simulink model "RudderActuatorChannel_control_arx"  (R2015a)
settings: Solver=ode4  StartTime=0.0  StopTime=2.999  FixedStep=sampleTime  MaxStep=1e-3  MinStep=1e-4
undefined symbols (not defined in the file or in its folder): Acv, Aleak1, Aleak2, Aleak3, Aleak4, Aleak5, Aleakext, Aleakint, Ap, Ap_seal, Ar_seal, As_ehsv, Bkp_seal, Bp1, C, Cd, ControlTopology, DeltaQ_ehsv, EHSV, EHSV_Step, EHSVFreqTest, EHSVTest, ent_air, frictionstribeck_velocity, i_ehsv, Imax, K2_ehsv, K3_ehsv, K_Supply1, Ka1, Kd, Ki, Ki_ehsv, Kp, Kr_ehsv, ksi_ehsv, Kst, Kst_Enable, Kw_ehsv, L0, Load_cmd, Lp_seal, Lr_seal, Max_Cmd, Max_Load_TED, Max_Load_TEU, Min_Cmd, Mp1, ON_OFF_hyst, P10, Pcvac, Pcvi, Pcvr, Ps0, Pt0, Ql_ehsv, R, Rate_Limit, Return_Pressure, Rho ... (+24)
undefined symbols (not defined in the file): dpLVDT, Kd_N, ramLVDT, StateControl, xvLVDT
libraries: simulink x3
(part 2 of 2)

== system RudderActuatorChannel_control_arx/Actuation System/Actuator/Valves Dynamics/EHSV/EHSV 1st Stage ==
  i : Inport
  Add : Sum  Inputs=|+-
  Armature flapper : TransferFcn  Numerator=[1/Kr_ehsv]  Denominator=[1/(w_n_ehsv^2) 2*ksi_ehsv/w_n_ehsv 1]
  EHSV 1st stage test : TransferFcn  Numerator=[.001852*730^2]  Denominator=[1 2*0.4*730 730^2]
  Feedback wire : Gain  Gain=Kw_ehsv
  Flapper displacement at nozzles : Saturate  UpperLimit=xf_ehsv  LowerLimit=-xf_ehsv
  Hydraulic Amplifier : Gain  Gain=K2_ehsv
  "Hydraulic Amplifier Differential flow " : Saturate  UpperLimit=DeltaQ_ehsv  LowerLimit=-DeltaQ_ehsv
  Scope : Scope  NumInputPorts=2
      settings: TimeRange=2.999  YMin=-5~-5  YMax=5~5  SaveName=ScopeData3
  Servovalve control flow : Saturate  UpperLimit=Ql_ehsv  LowerLimit=-Ql_ehsv
  Spool : TransferFcn  Denominator=[As_ehsv 0]
  Spool displacement : Saturate  UpperLimit=xs_ehsv  LowerLimit=-xs_ehsv
  Spool Flow Gain : Gain  Gain=K3_ehsv
  Terminator : Terminator
  Torque motor : Gain  Gain=Ki_ehsv
  Torque motor current : Saturate  UpperLimit=i_ehsv  LowerLimit=-i_ehsv
  Xv : Outport
  wires:
  Torque motor/1 -> Add/1
  Feedback wire/1 -> Add/2
  i/1 -> EHSV 1st stage test/1, Torque motor current/1
  Armature flapper/1 -> Flapper displacement at nozzles/1
  Spool/1 -> Scope/1, Spool displacement/1
  Hydraulic Amplifier/1 -> "Hydraulic Amplifier Differential flow "/1
  Add/1 -> Armature flapper/1
  Flapper displacement at nozzles/1 -> Hydraulic Amplifier/1
  "Hydraulic Amplifier Differential flow "/1 -> Spool/1
  Spool displacement/1 -> Spool Flow Gain/1, Xv/1, Feedback wire/1
  Torque motor current/1 -> Torque motor/1
  Spool Flow Gain/1 -> Servovalve control flow/1
  Servovalve control flow/1 -> Terminator/1
  EHSV 1st stage test/1 -> Scope/2

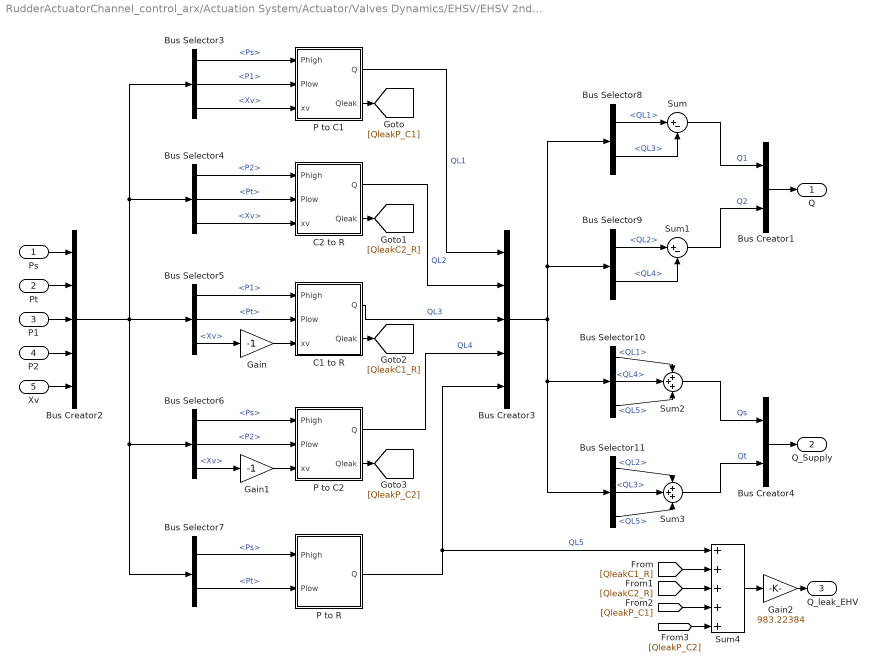
== system RudderActuatorChannel_control_arx/Actuation System/Actuator/Valves Dynamics/EHSV/EHSV 2nd Stage ==
  Ps : Inport
  Pt : Inport  Port=2
  P1 : Inport  Port=3
  P2 : Inport  Port=4
  Xv : Inport  Port=5
  Bus Creator1 : BusCreator  Inputs=2
  Bus Creator2 : BusCreator  Inputs=5
  Bus Creator3 : BusCreator  Inputs=5
  Bus Creator4 : BusCreator  Inputs=2
  Bus Selector10 : BusSelector  OutputSignals=QL1,QL4,QL5
  Bus Selector11 : BusSelector  OutputSignals=QL2,QL3,QL5
  Bus Selector3 : BusSelector  OutputSignals=Ps,P1,Xv
  Bus Selector4 : BusSelector  OutputSignals=P2,Pt,Xv
  Bus Selector5 : BusSelector  OutputSignals=P1,Pt,Xv
  Bus Selector6 : BusSelector  OutputSignals=Ps,P2,Xv
  Bus Selector7 : BusSelector  OutputSignals=Ps,Pt
  Bus Selector8 : BusSelector  OutputSignals=QL1,QL3
  Bus Selector9 : BusSelector  OutputSignals=QL2,QL4
  C1 to R : Subsystem
  C2 to R : Subsystem
  Gain : Gain  Gain=-1
  Gain1 : Gain  Gain=-1
  Gain2 : Gain  Gain=983.22384
  P to C1 : Subsystem
  P to C2 : Subsystem
  P to R : Subsystem
  Sum : Sum  Inputs=|+-
  Sum1 : Sum  Inputs=|+-
  Sum2 : Sum  Inputs=+++
  Sum3 : Sum  Inputs=+++
  Sum4 : Sum  Inputs=+++++
  Q : Outport
  Q_Supply : Outport  Port=2
  Q_leak_EHV : Outport  Port=3
  wires:
  Bus Creator1/1 -> Q/1
  Bus Selector3/1 -> P to C1/1(Phigh)  "<Ps>"
  Bus Selector3/2 -> P to C1/2(Plow)  "<P1>"
  Bus Selector3/3 -> P to C1/3(xv)  "<Xv>"
  Bus Selector4/1 -> C2 to R/1(Phigh)  "<P2>"
  Bus Selector4/2 -> C2 to R/2(Plow)  "<Pt>"
  Bus Selector4/3 -> C2 to R/3(xv)  "<Xv>"
  Bus Selector5/3 -> Gain/1  "<Xv>"
  Bus Selector6/1 -> P to C2/1(Phigh)  "<Ps>"
  Bus Selector6/2 -> P to C2/2(Plow)  "<P2>"
  Bus Selector6/3 -> Gain1/1  "<Xv>"
  Bus Selector7/1 -> P to R/1(Phigh)  "<Ps>"
  Bus Selector7/2 -> P to R/2(Plow)  "<Pt>"
  Bus Selector5/1 -> C1 to R/1(Phigh)  "<P1>"
  Bus Selector5/2 -> C1 to R/2(Plow)  "<Pt>"
  P to C1/1(Q) -> Bus Creator3/1  "QL1"
  C2 to R/1(Q) -> Bus Creator3/2  "QL2"
  C1 to R/1(Q) -> Bus Creator3/3  "QL3"
  P to C2/1(Q) -> Bus Creator3/4  "QL4"
  P to R/1(Q) -> Sum4/1, Bus Creator3/5  "QL5"
  Bus Creator2/1 -> Bus Selector5/1, Bus Selector3/1, Bus Selector4/1, Bus Selector7/1, Bus Selector6/1
  Bus Selector8/1 -> Sum/1  "<QL1>"
  Bus Selector8/2 -> Sum/2  "<QL3>"
  Bus Selector9/1 -> Sum1/1  "<QL2>"
  Bus Selector9/2 -> Sum1/2  "<QL4>"
  Bus Selector10/1 -> Sum2/1  "<QL1>"
  Bus Selector10/2 -> Sum2/2  "<QL4>"
  Bus Selector10/3 -> Sum2/3  "<QL5>"
  Bus Selector11/1 -> Sum3/1  "<QL2>"
  Bus Selector11/2 -> Sum3/2  "<QL3>"
  Bus Selector11/3 -> Sum3/3  "<QL5>"
  Bus Creator4/1 -> Q_Supply/1
  Bus Creator3/1 -> Bus Selector8/1, Bus Selector9/1, Bus Selector11/1, Bus Selector10/1
  Sum/1 -> Bus Creator1/1  "Q1"
  Sum1/1 -> Bus Creator1/2  "Q2"
  Sum2/1 -> Bus Creator4/1  "Qs"
  Sum3/1 -> Bus Creator4/2  "Qt"
  Ps/1 -> Bus Creator2/1
  Pt/1 -> Bus Creator2/2
  P1/1 -> Bus Creator2/3
  P2/1 -> Bus Creator2/4
  Xv/1 -> Bus Creator2/5
  Gain/1 -> C1 to R/3(xv)
  Gain1/1 -> P to C2/3(xv)
  Sum4/1 -> Gain2/1
  P to C1/2(Qleak) -> [QleakP_C1]
  C2 to R/2(Qleak) -> [QleakC2_R]
  C1 to R/2(Qleak) -> [QleakC1_R]
  P to C2/2(Qleak) -> [QleakP_C2]
  [QleakC1_R] -> Sum4/2
  [QleakC2_R] -> Sum4/3
  [QleakP_C2] -> Sum4/5
  [QleakP_C1] -> Sum4/4
  Gain2/1 -> Q_leak_EHV/1

== system RudderActuatorChannel_control_arx/Actuation System/Actuator/Valves Dynamics/EHSV/EHSV Test ==
  In1 : Inport
  Constant1 : Constant  Value=EHSVTest.Enable
  Constant3 : Constant  Value=1500
  EHVS freq test Selector1 : MultiPortSwitch
  Out1 : Outport
  wires:
  Constant1/1 -> EHVS freq test Selector1/1
  EHVS freq test Selector1/1 -> Out1/1
  In1/1 -> EHVS freq test Selector1/4, EHVS freq test Selector1/2
  Constant3/1 -> EHVS freq test Selector1/3

== system RudderActuatorChannel_control_arx/Actuation System/Actuator/Valves Dynamics/EHSV/EHSV Test1 ==
  In1 : Inport
  Constant1 : Constant  Value=EHSVTest.Enable
  Constant3 : Constant  Value=1500
  EHVS freq test Selector1 : MultiPortSwitch
  Out1 : Outport
  wires:
  Constant1/1 -> EHVS freq test Selector1/1
  EHVS freq test Selector1/1 -> Out1/1
  In1/1 -> EHVS freq test Selector1/4, EHVS freq test Selector1/2
  Constant3/1 -> EHVS freq test Selector1/3

== system RudderActuatorChannel_control_arx/Actuation System/Actuator/Valves Dynamics/EHSV/EHSV Test2 ==
  In1 : Inport
  Constant1 : Constant  Value=EHSVTest.Enable
  Constant3 : Constant  Value=3000
  EHVS freq test Selector1 : MultiPortSwitch
  Out1 : Outport
  wires:
  Constant1/1 -> EHVS freq test Selector1/1
  EHVS freq test Selector1/1 -> Out1/1
  In1/1 -> EHVS freq test Selector1/4, EHVS freq test Selector1/2
  Constant3/1 -> EHVS freq test Selector1/3

== system RudderActuatorChannel_control_arx/Actuation System/Actuator/Valves Dynamics/EHSV/EHSV Test3 ==
  In1 : Inport
  Constant1 : Constant  Value=EHSVTest.Enable
  Constant3 : Constant  Value=0
  EHVS freq test Selector1 : MultiPortSwitch
  Out1 : Outport
  wires:
  Constant1/1 -> EHVS freq test Selector1/1
  EHVS freq test Selector1/1 -> Out1/1
  In1/1 -> EHVS freq test Selector1/4, EHVS freq test Selector1/2
  Constant3/1 -> EHVS freq test Selector1/3

== system RudderActuatorChannel_control_arx/Actuation System/Actuator/Valves Dynamics/EHSV/EHSV input ==
  CurrentCmd : Inport
  Constant : Constant  Value=EHSVTest.Enable
  EHSV Freq Test : Sin  Amplitude=EHSVFreqTest.Sine.Amplitude  Bias=EHSVFreqTest.Sine.Bias  Frequency=EHSVFreqTest.Sine.Frequency  SampleTime=0
  EHVS freq test Selector : MultiPortSwitch
  Step : Step  Time=EHSV.Step.Time  After=EHSV.Step.Value  SampleTime=0
  EHSV_current : Outport
  wires:
  Constant/1 -> EHVS freq test Selector/1
  EHSV Freq Test/1 -> EHVS freq test Selector/3
  Step/1 -> EHVS freq test Selector/4
  EHVS freq test Selector/1 -> EHSV_current/1  "EHSV_current_cmd"
  CurrentCmd/1 -> EHVS freq test Selector/2

== system RudderActuatorChannel_control_arx/Actuation System/Actuator/Valves Dynamics/Inlet Check Valve/Inlet Check Valve Flow ==
  P1 : Inport
  P2 : Inport  Port=2
  Abs : Abs
  Constant : Constant  Value=Acv*sqrt(2/Rho)
  Constant1 : Constant  Value=Pcvi
  Gain : Gain  Gain=Cd/Pcvi
  Math Function : Math  Operator=sqrt  SaturateOnIntegerOverflow=on
  Product : Product  RndMeth=Zero
  Product1 : Product  RndMeth=Zero
  Product2 : Product  RndMeth=Zero
  Saturation : Saturate  UpperLimit=Cd  LowerLimit=0
  Sign : Signum
  Sum : Sum  Inputs=|+-
  Sum1 : Sum  Inputs=|+-
  Q : Outport
  wires:
  P1/1 -> Sum/1
  P2/1 -> Sum/2
  Sum/1 -> Sum1/1, Abs/1, Sign/1
  Constant1/1 -> Sum1/2
  Sum1/1 -> Gain/1
  Gain/1 -> Saturation/1
  Saturation/1 -> Product/1
  Constant/1 -> Product/2
  Abs/1 -> Math Function/1
  Sign/1 -> Product1/1
  Math Function/1 -> Product1/2
  Product1/1 -> Product2/1
  Product/1 -> Product2/2
  Product2/1 -> Q/1

== system RudderActuatorChannel_control_arx/Actuation System/Actuator/Valves Dynamics/Return Check Valve/Return Check Valve Flow ==
  P1 : Inport
  P2 : Inport  Port=2
  Abs : Abs
  Constant : Constant  Value=Acv*sqrt(2/Rho)
  Constant1 : Constant  Value=Pcvr
  Gain : Gain  Gain=Cd/Pcvr
  Math Function : Math  Operator=sqrt  SaturateOnIntegerOverflow=on
  Product : Product  RndMeth=Zero
  Product1 : Product  RndMeth=Zero
  Product2 : Product  RndMeth=Zero
  Saturation : Saturate  UpperLimit=Cd  LowerLimit=0
  Sign : Signum
  Sum : Sum  Inputs=|-+
  Sum1 : Sum  Inputs=|+-
  Q : Outport
  wires:
  P1/1 -> Sum/1
  P2/1 -> Sum/2
  Sum/1 -> Sum1/1, Abs/1, Sign/1
  Constant1/1 -> Sum1/2
  Sum1/1 -> Gain/1
  Gain/1 -> Saturation/1
  Saturation/1 -> Product/1
  Constant/1 -> Product/2
  Abs/1 -> Math Function/1
  Sign/1 -> Product1/1
  Math Function/1 -> Product1/2
  Product1/1 -> Product2/1
  Product/1 -> Product2/2
  Product2/1 -> Q/1

== system RudderActuatorChannel_control_arx/Actuation System/Actuator/Cylinder Dynamics/Piston Dynamics/Seal Friction Force/Force friction 2 Rod backup + scrapper seal ==
  Pressure : Inport
  Ar : Gain  Gain=Ar_seal
  Fc+Fh2 : Sum
  Friction - O-ring compression1 : Lookup_n-D  BreakpointsForDimension1=[0,5,10,15,20,25]  BreakpointsForDimension2=[70,80,90]  IndexSearchMethod=Linear search  Table=reshape([0,0.3,0.65,0.97313,1.37,1.7,0,0.6,1.22,1.82,2.45,3.05,0,0.8,1.6,2.37,3.2,3.98],6,3)  RndMeth=Simplest  InputSameDT=on
  Friction - O-ring hydraulic pressure1 : Lookup_n-D  NumberOfTableDimensions=1  BreakpointsForDimension1=|  BreakpointsForDimension2=[70,80,90]  IndexSearchMethod=Linear search  Table=|  RndMeth=Simplest  InputSameDT=on
      BreakpointsForDimension1=|
      | [0
      | 500
      | 1000
      | 1500
      | 2000
      | 2500
      | 3000]
      Table=|
      | [0
      | 24.5
      | 37.5
      | 48
      | 58
      | 67
      | 72.1]
  Lr : Gain  Gain=Lr_seal
  Seal compression : Constant  Value=seal_compression
  Seal hardness : Constant  Value=seal_hardness
  Ffriction : Outport
  wires:
  Friction - O-ring compression1/1 -> Lr/1
  Lr/1 -> Fc+Fh2/2  "Fc"
  Pressure/1 -> Friction - O-ring hydraulic pressure1/1
  Friction - O-ring hydraulic pressure1/1 -> Ar/1
  Ar/1 -> Fc+Fh2/1  "Fh"
  Fc+Fh2/1 -> Ffriction/1
  Seal compression/1 -> [Seal_compression]
  [Seal_compression] -> Friction - O-ring compression1/1
  Seal hardness/1 -> [Seal_hardness]
  [Seal_hardness] -> Friction - O-ring compression1/2

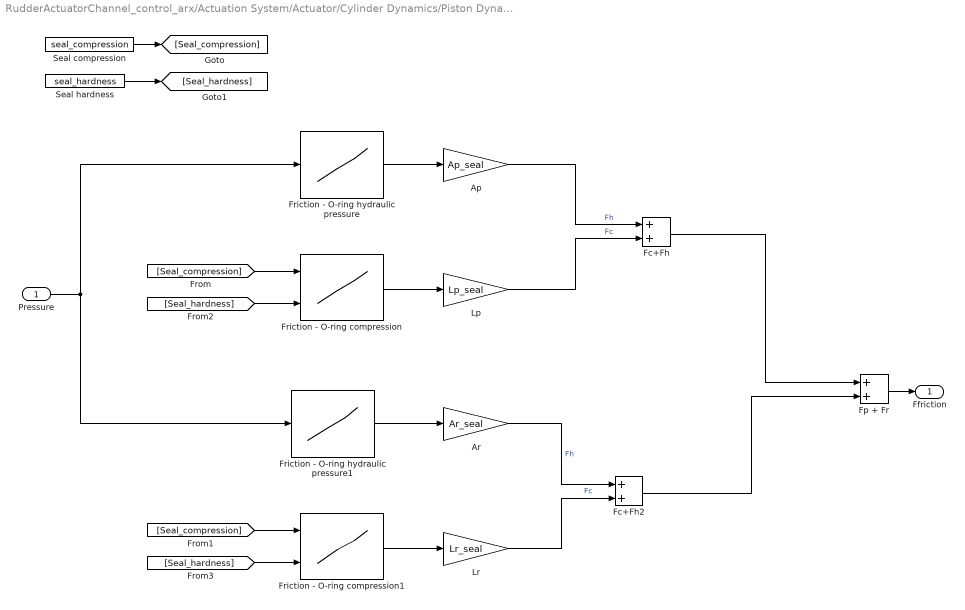
== system RudderActuatorChannel_control_arx/Actuation System/Actuator/Cylinder Dynamics/Piston Dynamics/Seal Friction Force/Force friction Piston+rod extension ==
  Pressure : Inport
  Ap : Gain  Gain=Ap_seal
  Ar : Gain  Gain=Ar_seal
  Fc+Fh : Sum
  Fc+Fh2 : Sum
  Fp + Fr : Sum
  Friction - O-ring compression : Lookup_n-D  BreakpointsForDimension1=[0,5,10,15,20,25]  BreakpointsForDimension2=[70,80,90]  IndexSearchMethod=Linear search  Table=reshape([0,0.3,0.65,0.97313,1.37,1.7,0,0.6,1.22,1.82,2.45,3.05,0,0.8,1.6,2.37,3.2,3.98],6,3)  RndMeth=Simplest  InputSameDT=on
  Friction - O-ring compression1 : Lookup_n-D  BreakpointsForDimension1=[0,5,10,15,20,25]  BreakpointsForDimension2=[70,80,90]  IndexSearchMethod=Linear search  Table=reshape([0,0.3,0.65,0.97313,1.37,1.7,0,0.6,1.22,1.82,2.45,3.05,0,0.8,1.6,2.37,3.2,3.98],6,3)  RndMeth=Simplest  InputSameDT=on
  Friction - O-ring hydraulic pressure : Lookup_n-D  NumberOfTableDimensions=1  BreakpointsForDimension1=|  BreakpointsForDimension2=[70,80,90]  IndexSearchMethod=Linear search  Table=|  RndMeth=Simplest  InputSameDT=on
      BreakpointsForDimension1=|
      | [0
      | 500
      | 1000
      | 1500
      | 2000
      | 2500
      | 3000]
      Table=|
      | [0
      | 24.5
      | 37.5
      | 48
      | 58
      | 67
      | 72.1]
  Friction - O-ring hydraulic pressure1 : Lookup_n-D  NumberOfTableDimensions=1  BreakpointsForDimension1=|  BreakpointsForDimension2=[70,80,90]  IndexSearchMethod=Linear search  Table=|  RndMeth=Simplest  InputSameDT=on
      BreakpointsForDimension1=|
      | [0
      | 500
      | 1000
      | 1500
      | 2000
      | 2500
      | 3000]
      Table=|
      | [0
      | 24.5
      | 37.5
      | 48
      | 58
      | 67
      | 72.1]
  Lp : Gain  Gain=Lp_seal
  Lr : Gain  Gain=Lr_seal
  Seal compression : Constant  Value=seal_compression
  Seal hardness : Constant  Value=seal_hardness
  Ffriction : Outport
  wires:
  Friction - O-ring compression/1 -> Lp/1
  Lp/1 -> Fc+Fh/2  "Fc"
  Friction - O-ring hydraulic pressure/1 -> Ap/1
  Ap/1 -> Fc+Fh/1  "Fh"
  Fp + Fr/1 -> Ffriction/1
  Friction - O-ring compression1/1 -> Lr/1
  Lr/1 -> Fc+Fh2/2  "Fc"
  Pressure/1 -> Friction - O-ring hydraulic pressure/1, Friction - O-ring hydraulic pressure1/1
  Friction - O-ring hydraulic pressure1/1 -> Ar/1
  Ar/1 -> Fc+Fh2/1  "Fh"
  Fc+Fh2/1 -> Fp + Fr/2
  Fc+Fh/1 -> Fp + Fr/1
  Seal compression/1 -> [Seal_compression]
  [Seal_compression] -> Friction - O-ring compression/1
  [Seal_compression] -> Friction - O-ring compression1/1
  Seal hardness/1 -> [Seal_hardness]
  [Seal_hardness] -> Friction - O-ring compression/2
  [Seal_hardness] -> Friction - O-ring compression1/2

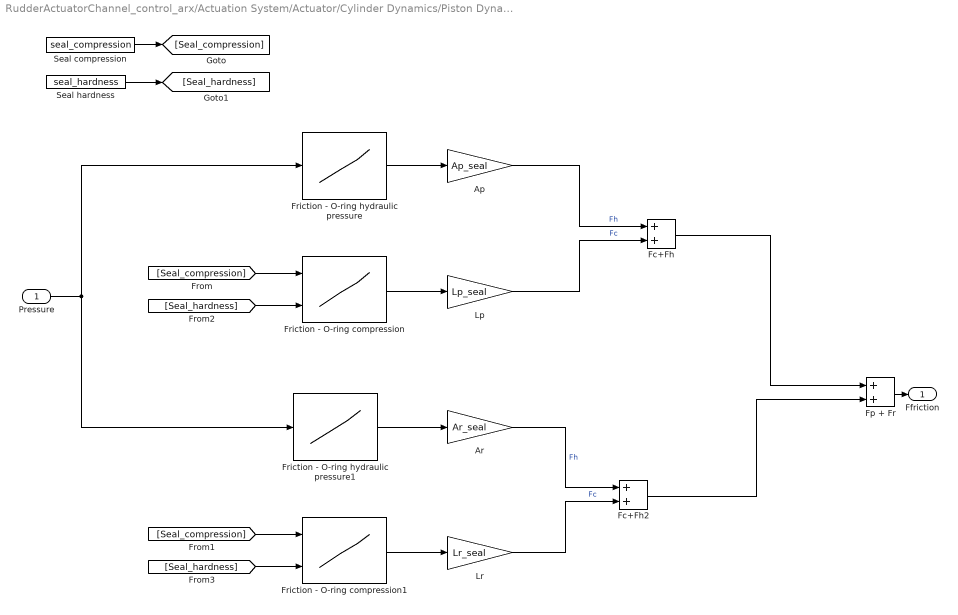
== system RudderActuatorChannel_control_arx/Actuation System/Actuator/Cylinder Dynamics/Piston Dynamics/Seal Friction Force/Force friction Piston+rod retraction ==
  Pressure : Inport
  Ap : Gain  Gain=Ap_seal
  Ar : Gain  Gain=Ar_seal
  Fc+Fh : Sum
  Fc+Fh2 : Sum
  Fp + Fr : Sum
  Friction - O-ring compression : Lookup_n-D  BreakpointsForDimension1=[0,5,10,15,20,25]  BreakpointsForDimension2=[70,80,90]  IndexSearchMethod=Linear search  Table=reshape([0,0.3,0.65,0.97313,1.37,1.7,0,0.6,1.22,1.82,2.45,3.05,0,0.8,1.6,2.37,3.2,3.98],6,3)  RndMeth=Simplest  InputSameDT=on
  Friction - O-ring compression1 : Lookup_n-D  BreakpointsForDimension1=[0,5,10,15,20,25]  BreakpointsForDimension2=[70,80,90]  IndexSearchMethod=Linear search  Table=reshape([0,0.3,0.65,0.97313,1.37,1.7,0,0.6,1.22,1.82,2.45,3.05,0,0.8,1.6,2.37,3.2,3.98],6,3)  RndMeth=Simplest  InputSameDT=on
  Friction - O-ring hydraulic pressure : Lookup_n-D  NumberOfTableDimensions=1  BreakpointsForDimension1=|  BreakpointsForDimension2=[70,80,90]  IndexSearchMethod=Linear search  Table=|  RndMeth=Simplest  InputSameDT=on
      BreakpointsForDimension1=|
      | [0
      | 500
      | 1000
      | 1500
      | 2000
      | 2500
      | 3000]
      Table=|
      | [0
      | 24.5
      | 37.5
      | 48
      | 58
      | 67
      | 72.1]
  Friction - O-ring hydraulic pressure1 : Lookup_n-D  NumberOfTableDimensions=1  BreakpointsForDimension1=|  BreakpointsForDimension2=[70,80,90]  IndexSearchMethod=Linear search  Table=|  RndMeth=Simplest  InputSameDT=on
      BreakpointsForDimension1=|
      | [0
      | 500
      | 1000
      | 1500
      | 2000
      | 2500
      | 3000]
      Table=|
      | [0
      | 24.5
      | 37.5
      | 48
      | 58
      | 67
      | 72.1]
  Lp : Gain  Gain=Lp_seal
  Lr : Gain  Gain=Lr_seal
  Seal compression : Constant  Value=seal_compression
  Seal hardness : Constant  Value=seal_hardness
  Ffriction : Outport
  wires:
  Friction - O-ring compression/1 -> Lp/1
  Lp/1 -> Fc+Fh/2  "Fc"
  Friction - O-ring hydraulic pressure/1 -> Ap/1
  Ap/1 -> Fc+Fh/1  "Fh"
  Fp + Fr/1 -> Ffriction/1
  Friction - O-ring compression1/1 -> Lr/1
  Lr/1 -> Fc+Fh2/2  "Fc"
  Pressure/1 -> Friction - O-ring hydraulic pressure/1, Friction - O-ring hydraulic pressure1/1
  Friction - O-ring hydraulic pressure1/1 -> Ar/1
  Ar/1 -> Fc+Fh2/1  "Fh"
  Fc+Fh2/1 -> Fp + Fr/2
  Fc+Fh/1 -> Fp + Fr/1
  Seal compression/1 -> [Seal_compression]
  [Seal_compression] -> Friction - O-ring compression/1
  [Seal_compression] -> Friction - O-ring compression1/1
  Seal hardness/1 -> [Seal_hardness]
  [Seal_hardness] -> Friction - O-ring compression/2
  [Seal_hardness] -> Friction - O-ring compression1/2

== system RudderActuatorChannel_control_arx/Actuation System/Actuator/Cylinder Dynamics/Piston Dynamics/Seal Friction Force/Stribeck effect ==
  Xp : Inport
  Abs : Abs
  Backlash : Backlash  BacklashWidth=.1
  Divide : Product  Inputs=*/
  Fcn : Fcn  Expr=exp(-u/frictionstribeck_velocity)
  Manual Switch : ManualSwitch  CurrentSetting=0
  Manual Switch1 : ManualSwitch  CurrentSetting=0
  Product : Product  RndMeth=Zero
  Stribeck factor : Outport
  wires:
  Xp/1 -> Manual Switch1/1, Backlash/1
  Abs/1 -> Divide/1, Fcn/1
  Fcn/1 -> Manual Switch/2, Product/2
  Divide/1 -> Product/1
  Product/1 -> Manual Switch/1
  Manual Switch/1 -> Stribeck factor/1
  Manual Switch1/1 -> Divide/2, Abs/1
  Backlash/1 -> Manual Switch1/2

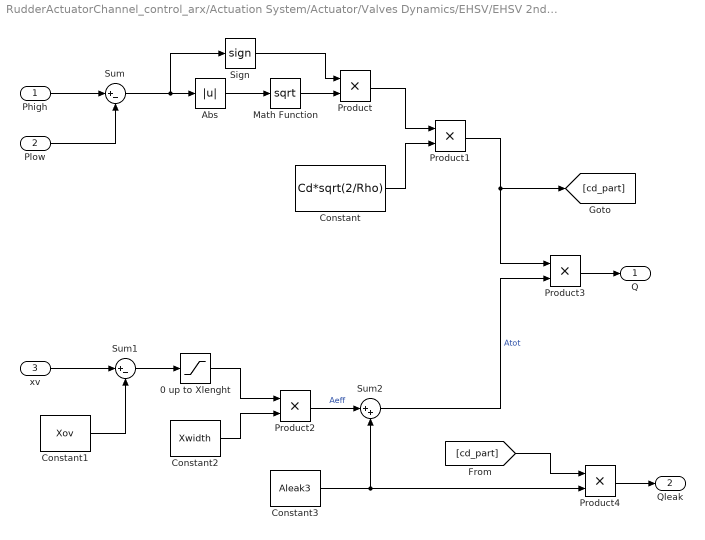
== system RudderActuatorChannel_control_arx/Actuation System/Actuator/Valves Dynamics/EHSV/EHSV 2nd Stage/C1 to R ==
  Phigh : Inport
  Plow : Inport  Port=2
  xv : Inport  Port=3
  0 up to Xlenght : Saturate  UpperLimit=Xlength  LowerLimit=0
  Abs : Abs
  Constant : Constant  Value=Cd*sqrt(2/Rho)
  Constant1 : Constant  Value=Xov
  Constant2 : Constant  Value=Xwidth
  Constant3 : Constant  Value=Aleak3
  Math Function : Math  Operator=sqrt  SaturateOnIntegerOverflow=on
  Product{,1..4} (5 alike) : Product  RndMeth=Zero
  Sign : Signum
  Sum : Sum  Inputs=|+-
  Sum1 : Sum  Inputs=|+-
  Sum2 : Sum  Inputs=|++
  Q : Outport
  Qleak : Outport  Port=2
  wires:
  Phigh/1 -> Sum/1
  Plow/1 -> Sum/2
  Sum/1 -> Abs/1, Sign/1
  Abs/1 -> Math Function/1
  Sign/1 -> Product/1
  Math Function/1 -> Product/2
  Constant/1 -> Product1/2
  Product/1 -> Product1/1
  xv/1 -> Sum1/1
  Constant1/1 -> Sum1/2
  Sum1/1 -> 0 up to Xlenght/1
  0 up to Xlenght/1 -> Product2/1
  Constant2/1 -> Product2/2
  Product2/1 -> Sum2/1  "Aeff"
  Constant3/1 -> Product4/2, Sum2/2
  Product1/1 -> [cd_part], Product3/1
  Sum2/1 -> Product3/2  "Atot"
  Product3/1 -> Q/1
  Product4/1 -> Qleak/1
  [cd_part] -> Product4/1

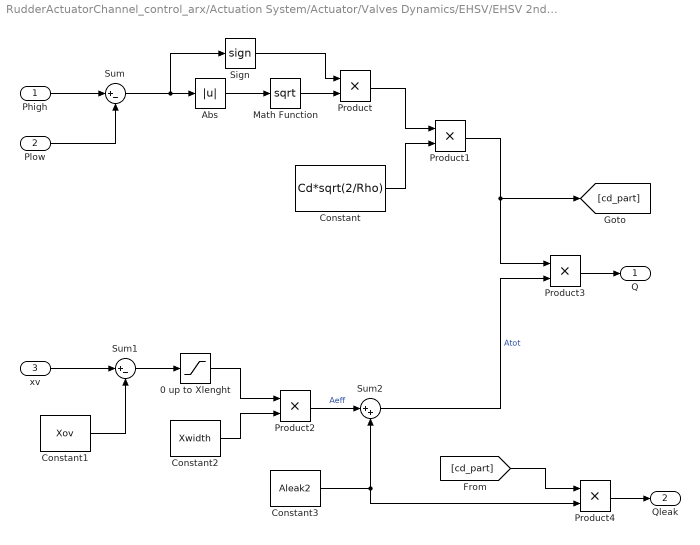
== system RudderActuatorChannel_control_arx/Actuation System/Actuator/Valves Dynamics/EHSV/EHSV 2nd Stage/C2 to R ==
  Phigh : Inport
  Plow : Inport  Port=2
  xv : Inport  Port=3
  0 up to Xlenght : Saturate  UpperLimit=Xlength  LowerLimit=0
  Abs : Abs
  Constant : Constant  Value=Cd*sqrt(2/Rho)
  Constant1 : Constant  Value=Xov
  Constant2 : Constant  Value=Xwidth
  Constant3 : Constant  Value=Aleak2
  Math Function : Math  Operator=sqrt  SaturateOnIntegerOverflow=on
  Product{,1..4} (5 alike) : Product  RndMeth=Zero
  Sign : Signum
  Sum : Sum  Inputs=|+-
  Sum1 : Sum  Inputs=|+-
  Sum2 : Sum  Inputs=|++
  Q : Outport
  Qleak : Outport  Port=2
  wires:
  Product3/1 -> Q/1
  Sum2/1 -> Product3/2  "Atot"
  Product1/1 -> [cd_part], Product3/1
  Product2/1 -> Sum2/1  "Aeff"
  Constant2/1 -> Product2/2
  0 up to Xlenght/1 -> Product2/1
  Sum1/1 -> 0 up to Xlenght/1
  Constant1/1 -> Sum1/2
  xv/1 -> Sum1/1
  Product/1 -> Product1/1
  Constant/1 -> Product1/2
  Math Function/1 -> Product/2
  Sign/1 -> Product/1
  Abs/1 -> Math Function/1
  Sum/1 -> Sign/1, Abs/1
  Plow/1 -> Sum/2
  Phigh/1 -> Sum/1
  Constant3/1 -> Product4/2, Sum2/2
  Product4/1 -> Qleak/1
  [cd_part] -> Product4/1

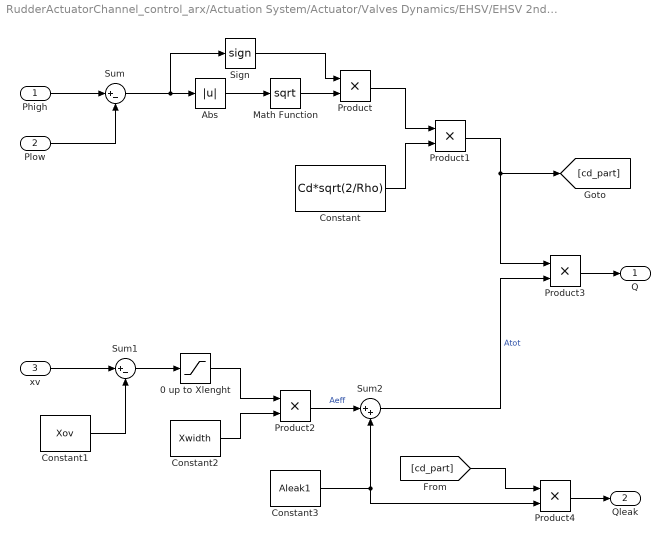
== system RudderActuatorChannel_control_arx/Actuation System/Actuator/Valves Dynamics/EHSV/EHSV 2nd Stage/P to C1 ==
  Phigh : Inport
  Plow : Inport  Port=2
  xv : Inport  Port=3
  0 up to Xlenght : Saturate  UpperLimit=Xlength  LowerLimit=0
  Abs : Abs
  Constant : Constant  Value=Cd*sqrt(2/Rho)
  Constant1 : Constant  Value=Xov
  Constant2 : Constant  Value=Xwidth
  Constant3 : Constant  Value=Aleak1
  Math Function : Math  Operator=sqrt  SaturateOnIntegerOverflow=on
  Product{,1..4} (5 alike) : Product  RndMeth=Zero
  Sign : Signum
  Sum : Sum  Inputs=|+-
  Sum1 : Sum  Inputs=|+-
  Sum2 : Sum  Inputs=|++
  Q : Outport
  Qleak : Outport  Port=2
  wires:
  Phigh/1 -> Sum/1
  Plow/1 -> Sum/2
  Sum/1 -> Abs/1, Sign/1
  Abs/1 -> Math Function/1
  Sign/1 -> Product/1
  Math Function/1 -> Product/2
  Constant/1 -> Product1/2
  Product/1 -> Product1/1
  xv/1 -> Sum1/1
  Constant1/1 -> Sum1/2
  Sum1/1 -> 0 up to Xlenght/1
  0 up to Xlenght/1 -> Product2/1
  Constant2/1 -> Product2/2
  Product2/1 -> Sum2/1  "Aeff"
  Constant3/1 -> Sum2/2, Product4/2
  Product1/1 -> [cd_part], Product3/1
  Sum2/1 -> Product3/2  "Atot"
  Product3/1 -> Q/1
  Product4/1 -> Qleak/1
  [cd_part] -> Product4/1

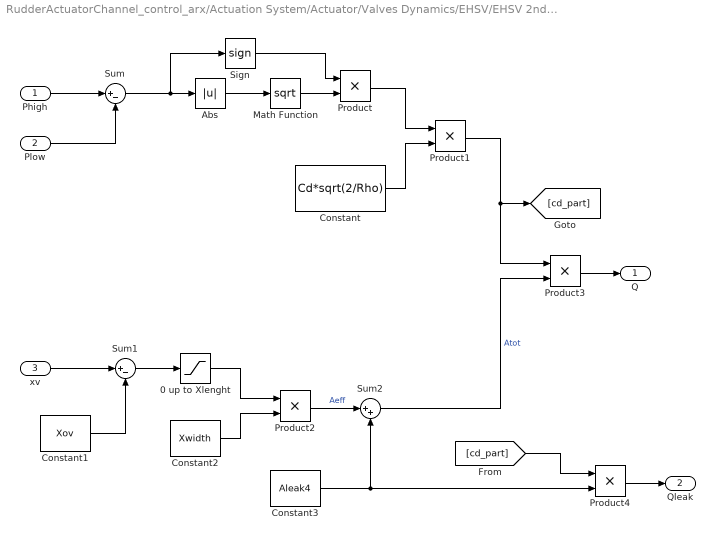
== system RudderActuatorChannel_control_arx/Actuation System/Actuator/Valves Dynamics/EHSV/EHSV 2nd Stage/P to C2 ==
  Phigh : Inport
  Plow : Inport  Port=2
  xv : Inport  Port=3
  0 up to Xlenght : Saturate  UpperLimit=Xlength  LowerLimit=0
  Abs : Abs
  Constant : Constant  Value=Cd*sqrt(2/Rho)
  Constant1 : Constant  Value=Xov
  Constant2 : Constant  Value=Xwidth
  Constant3 : Constant  Value=Aleak4
  Math Function : Math  Operator=sqrt  SaturateOnIntegerOverflow=on
  Product{,1..4} (5 alike) : Product  RndMeth=Zero
  Sign : Signum
  Sum : Sum  Inputs=|+-
  Sum1 : Sum  Inputs=|+-
  Sum2 : Sum  Inputs=|++
  Q : Outport
  Qleak : Outport  Port=2
  wires:
  Product3/1 -> Q/1
  Sum2/1 -> Product3/2  "Atot"
  Product1/1 -> [cd_part], Product3/1
  Product2/1 -> Sum2/1  "Aeff"
  Constant2/1 -> Product2/2
  0 up to Xlenght/1 -> Product2/1
  Sum1/1 -> 0 up to Xlenght/1
  Constant1/1 -> Sum1/2
  xv/1 -> Sum1/1
  Product/1 -> Product1/1
  Constant/1 -> Product1/2
  Math Function/1 -> Product/2
  Sign/1 -> Product/1
  Abs/1 -> Math Function/1
  Sum/1 -> Sign/1, Abs/1
  Plow/1 -> Sum/2
  Phigh/1 -> Sum/1
  Constant3/1 -> Sum2/2, Product4/2
  Product4/1 -> Qleak/1
  [cd_part] -> Product4/1

== system RudderActuatorChannel_control_arx/Actuation System/Actuator/Valves Dynamics/EHSV/EHSV 2nd Stage/P to R ==
  Phigh : Inport
  Plow : Inport  Port=2
  Abs : Abs
  Constant : Constant  Value=Cd*sqrt(2/Rho)
  Constant3 : Constant  Value=Aleak5
  Math Function : Math  Operator=sqrt  SaturateOnIntegerOverflow=on
  Product : Product  RndMeth=Zero
  Product1 : Product  RndMeth=Zero
  Product3 : Product  RndMeth=Zero
  Sign : Signum
  Sum : Sum  Inputs=|+-
  Q : Outport
  wires:
  Phigh/1 -> Sum/1
  Plow/1 -> Sum/2
  Sum/1 -> Abs/1, Sign/1
  Abs/1 -> Math Function/1
  Sign/1 -> Product/1
  Math Function/1 -> Product/2
  Constant/1 -> Product1/2
  Product/1 -> Product1/1
  Constant3/1 -> Product3/2  "Atot"
  Product1/1 -> Product3/1
  Product3/1 -> Q/1
